simulink model "racing_modes_R2022a"  (R2022a)
settings: Solver=FixedStepAuto  StartTime=0.0  StopTime=10.0  RelTol=1e-3
libraries: simulink x1
settings Model: Creator=no  LastModifiedBy=joser
settings OptimizationCC: DefaultParameterBehavior=Inlined
settings ModelReferenceCC: EnableRefExpFcnMdlSchedulingChecks=off
settings RTWCC: Description=INTECRIO Real-Time Target  SystemTargetFile=irt.tlc  TemplateMakefile=irt_default_tmf
settings STFCustomTargetCC: TargetLangStandard=C99 (ISO)  UtilityFuncGeneration=Shared location  MatFileLogging=on  SystemTargetFile=irt.tlc
settings GRTTargetCC: UtilityFuncGeneration=Shared location  ParMdlRefBuildCompliant=off  CompOptLevelCompliant=off  ConcurrentExecutionCompliant=off  CombineOutputUpdateFcns=off  CPPClassGenCompliant=off  GRTInterface=on  UseToolchainInfoCompliant=off  GenerateASAP2=on

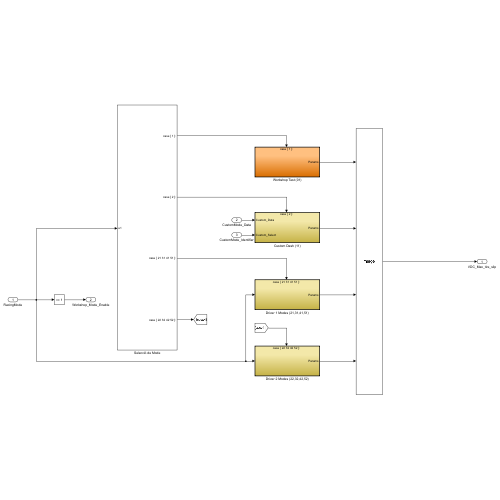
[thumbnail: Simulink's stored preview of the top-level diagram]
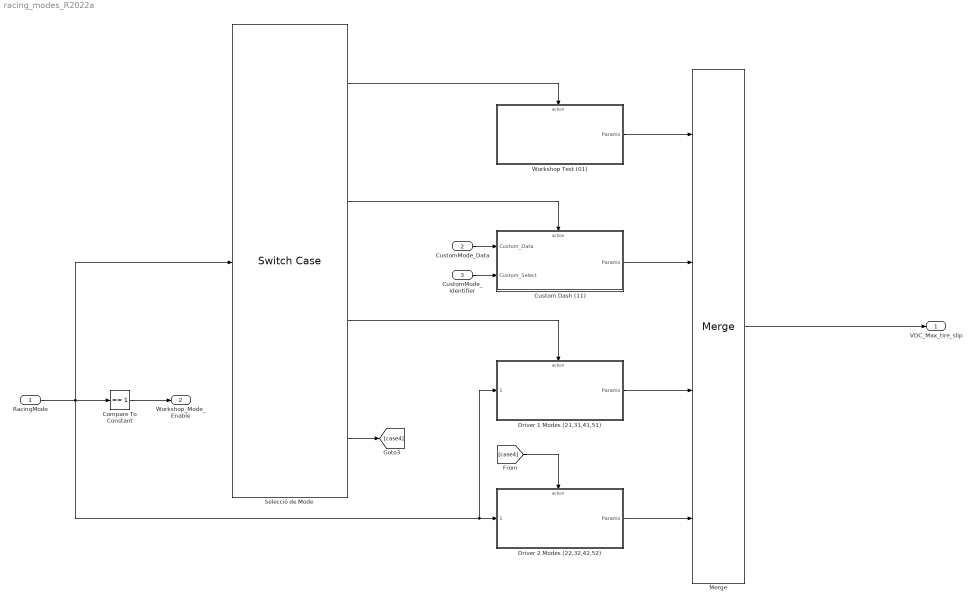
== system racing_modes_R2022a ==
  RacingMode : Inport  OutDataTypeStr=uint8
  CustomMode_Data : Inport  Port=2
  CustomMode_Identifier : Inport  Port=3
  Compare To Constant : simulink/Logic and Bit Operations/Compare To Constant  relop===  const=1  OutDataTypeStr=boolean
  Custom Dash (11) : Subsystem  TreatAsAtomicUnit=on
  Driver 1 Modes (21,31,41,51) : Subsystem  TreatAsAtomicUnit=on
  Driver 2 Modes (22,32,42,52) : Subsystem  TreatAsAtomicUnit=on
  Merge : Merge  Inputs=4
  Selecció de Mode : SwitchCase  CaseConditions={01, 2, [21,31,41,51], [22,32,42,52]}  ShowDefaultCase=off
  Workshop Test (01) : Subsystem  TreatAsAtomicUnit=on
  VDC_Max_tire_slip : Outport
  Workshop_Mode_Enable : Outport  Port=2
  wires:
  CustomMode_Identifier/1 -> Custom Dash (11)/2(Custom_Select)
  Custom Dash (11)/1(Params) -> Merge/2
  RacingMode/1 -> Driver 1 Modes (21,31,41,51)/1(" "), Driver 2 Modes (22,32,42,52)/1(" "), Compare To Constant/1, Selecció de Mode/1
  Workshop Test (01)/1(Params) -> Merge/1
  CustomMode_Data/1 -> Custom Dash (11)/1(Custom_Data)
  Driver 1 Modes (21,31,41,51)/1(Params) -> Merge/3
  Driver 2 Modes (22,32,42,52)/1(Params) -> Merge/4
  Selecció de Mode/4 -> [case4]
  [case4] -> Driver 2 Modes (22,32,42,52)/Action
  Selecció de Mode/1 -> Workshop Test (01)/Action
  Selecció de Mode/2 -> Custom Dash (11)/Action
  Selecció de Mode/3 -> Driver 1 Modes (21,31,41,51)/Action
  Merge/1 -> VDC_Max_tire_slip/1
  Compare To Constant/1 -> Workshop_Mode_Enable/1

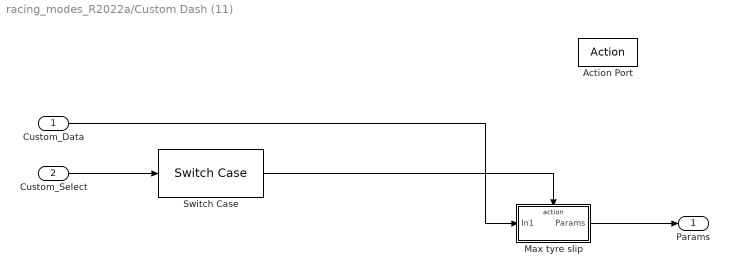
== system racing_modes_R2022a/Custom Dash (11) ==
  Custom_Data : Inport
  Custom_Select : Inport  Port=2
  Action Port : ActionPort  ActionPortLabel=case [ 2 ]:
  Max tyre slip : Subsystem  TreatAsAtomicUnit=on
  Switch Case : SwitchCase  ShowDefaultCase=off
  Params : Outport  VectorParamsAs1DForOutWhenUnconnected=off
  wires:
  Custom_Select/1 -> Switch Case/1
  Custom_Data/1 -> Max tyre slip/1(In1)
  Switch Case/1 -> Max tyre slip/Action
  Max tyre slip/1(Params) -> Params/1

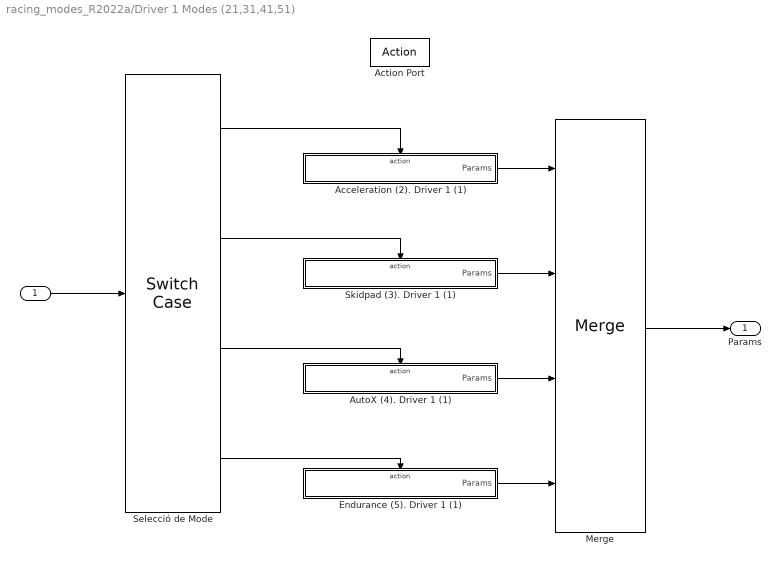
== system racing_modes_R2022a/Driver 1 Modes (21,31,41,51) ==
  " " : Inport  OutDataTypeStr=uint8
  Action Port : ActionPort  ActionPortLabel=case [ 21 31 41 51 ]:
  "Acceleration (2). Driver 1 (1) " : Subsystem  TreatAsAtomicUnit=on
  AutoX (4). Driver 1 (1) : Subsystem  TreatAsAtomicUnit=on
  Endurance (5). Driver 1 (1) : Subsystem  TreatAsAtomicUnit=on
  Merge : Merge  Inputs=4
  Selecció de Mode : SwitchCase  CaseConditions={21,31,41,51}  ShowDefaultCase=off
  Skidpad (3). Driver 1 (1) : Subsystem  TreatAsAtomicUnit=on
  Params : Outport  VectorParamsAs1DForOutWhenUnconnected=off
  wires:
  Merge/1 -> Params/1
  " "/1 -> Selecció de Mode/1
  Selecció de Mode/4 -> Endurance (5). Driver 1 (1)/Action
  Selecció de Mode/3 -> AutoX (4). Driver 1 (1)/Action
  Selecció de Mode/2 -> Skidpad (3). Driver 1 (1)/Action
  Selecció de Mode/1 -> "Acceleration (2). Driver 1 (1) "/Action
  "Acceleration (2). Driver 1 (1) "/1(Params) -> Merge/1
  Skidpad (3). Driver 1 (1)/1(Params) -> Merge/2
  AutoX (4). Driver 1 (1)/1(Params) -> Merge/3
  Endurance (5). Driver 1 (1)/1(Params) -> Merge/4

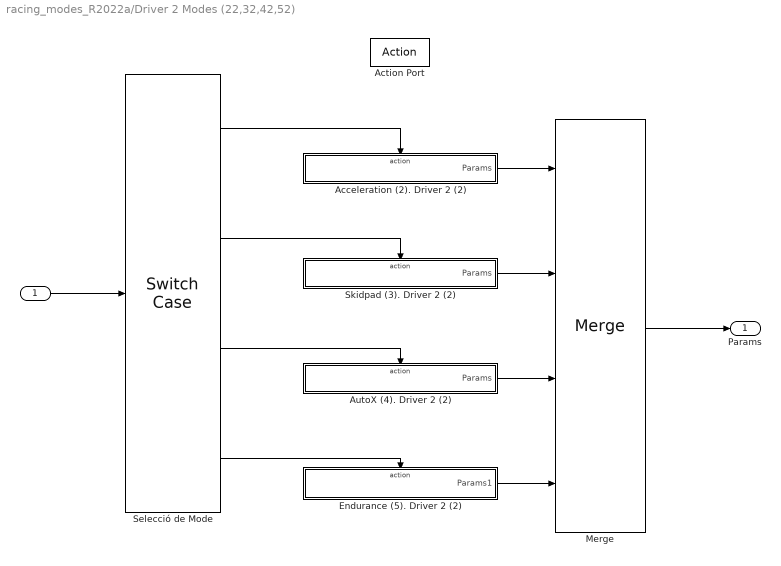
== system racing_modes_R2022a/Driver 2 Modes (22,32,42,52) ==
  " " : Inport  OutDataTypeStr=uint8
  Action Port : ActionPort  ActionPortLabel=case [ 22 32 42 52 ]:
  "Acceleration (2). Driver 2 (2) " : Subsystem  TreatAsAtomicUnit=on
  AutoX (4). Driver 2 (2) : Subsystem  TreatAsAtomicUnit=on
  Endurance (5). Driver 2 (2) : Subsystem  TreatAsAtomicUnit=on
  Merge : Merge  Inputs=4
  Selecció de Mode : SwitchCase  CaseConditions={22,32,42,52}  ShowDefaultCase=off
  Skidpad (3). Driver 2 (2) : Subsystem  TreatAsAtomicUnit=on
  Params : Outport  VectorParamsAs1DForOutWhenUnconnected=off
  wires:
  Merge/1 -> Params/1
  " "/1 -> Selecció de Mode/1
  Selecció de Mode/4 -> Endurance (5). Driver 2 (2)/Action
  Selecció de Mode/3 -> AutoX (4). Driver 2 (2)/Action
  Selecció de Mode/2 -> Skidpad (3). Driver 2 (2)/Action
  Selecció de Mode/1 -> "Acceleration (2). Driver 2 (2) "/Action
  "Acceleration (2). Driver 2 (2) "/1(Params) -> Merge/1
  Skidpad (3). Driver 2 (2)/1(Params) -> Merge/2
  AutoX (4). Driver 2 (2)/1(Params) -> Merge/3
  Endurance (5). Driver 2 (2)/1(Params1) -> Merge/4

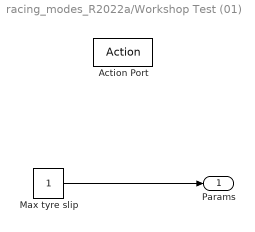
== system racing_modes_R2022a/Workshop Test (01) ==
  Action Port : ActionPort  ActionPortLabel=case [ 1 ]:
  Max tyre slip : Constant
  Params : Outport  VectorParamsAs1DForOutWhenUnconnected=off
  wires:
  Max tyre slip/1 -> Params/1

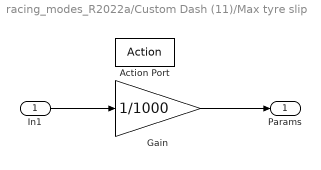
== system racing_modes_R2022a/Custom Dash (11)/Max tyre slip ==
  In1 : Inport
  Action Port : ActionPort
  Gain : Gain  Gain=1/1000
  Params : Outport  VectorParamsAs1DForOutWhenUnconnected=off
  wires:
  In1/1 -> Gain/1
  Gain/1 -> Params/1

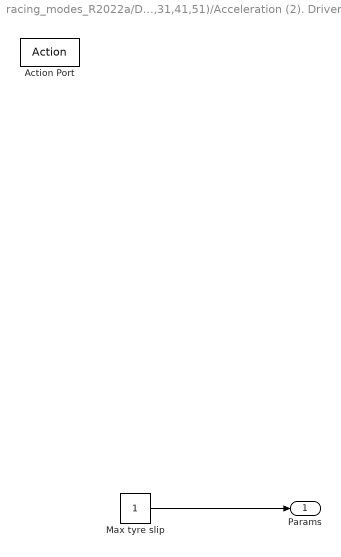
== system racing_modes_R2022a/Driver 1 Modes (21,31,41,51)/Acceleration (2). Driver 1 (1)  ==
  Action Port : ActionPort
  Max tyre slip : Constant
  Params : Outport  VectorParamsAs1DForOutWhenUnconnected=off
  wires:
  Max tyre slip/1 -> Params/1

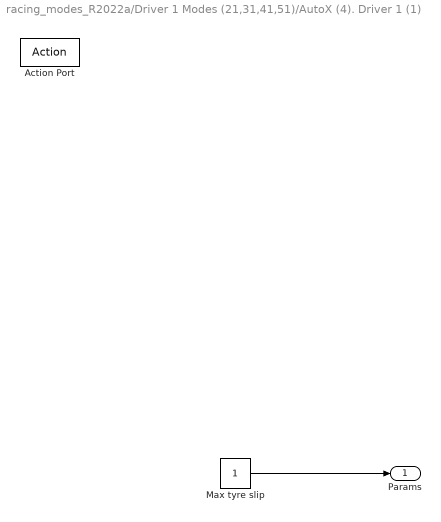
== system racing_modes_R2022a/Driver 1 Modes (21,31,41,51)/AutoX (4). Driver 1 (1) ==
  Action Port : ActionPort
  Max tyre slip : Constant
  Params : Outport  VectorParamsAs1DForOutWhenUnconnected=off
  wires:
  Max tyre slip/1 -> Params/1

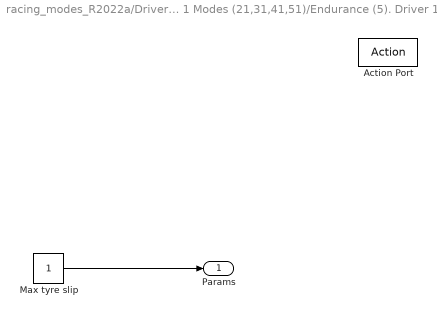
== system racing_modes_R2022a/Driver 1 Modes (21,31,41,51)/Endurance (5). Driver 1 (1) ==
  Action Port : ActionPort
  Max tyre slip : Constant
  Params : Outport  VectorParamsAs1DForOutWhenUnconnected=off
  wires:
  Max tyre slip/1 -> Params/1

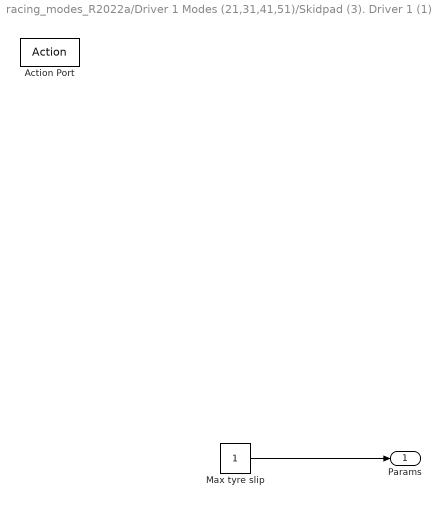
== system racing_modes_R2022a/Driver 1 Modes (21,31,41,51)/Skidpad (3). Driver 1 (1) ==
  Action Port : ActionPort  ActionPortLabel=case [ 31 ]:
  Max tyre slip : Constant
  Params : Outport  VectorParamsAs1DForOutWhenUnconnected=off
  wires:
  Max tyre slip/1 -> Params/1

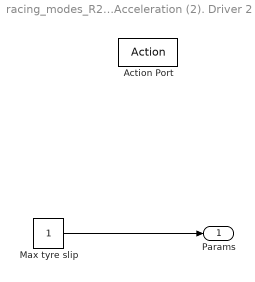
== system racing_modes_R2022a/Driver 2 Modes (22,32,42,52)/Acceleration (2). Driver 2 (2)  ==
  Action Port : ActionPort
  Max tyre slip : Constant
  Params : Outport  VectorParamsAs1DForOutWhenUnconnected=off
  wires:
  Max tyre slip/1 -> Params/1

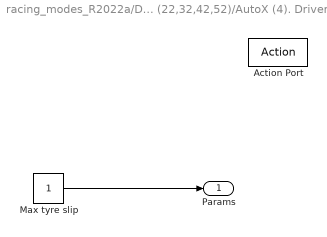
== system racing_modes_R2022a/Driver 2 Modes (22,32,42,52)/AutoX (4). Driver 2 (2) ==
  Action Port : ActionPort
  Max tyre slip : Constant
  Params : Outport  VectorParamsAs1DForOutWhenUnconnected=off
  wires:
  Max tyre slip/1 -> Params/1

== system racing_modes_R2022a/Driver 2 Modes (22,32,42,52)/Endurance (5). Driver 2 (2) ==
  Action Port : ActionPort
  Max tyre slip1 : Constant
  Params1 : Outport  VectorParamsAs1DForOutWhenUnconnected=off
  wires:
  Max tyre slip1/1 -> Params1/1

== system racing_modes_R2022a/Driver 2 Modes (22,32,42,52)/Skidpad (3). Driver 2 (2) ==
  Action Port : ActionPort  ActionPortLabel=case [ 32 ]:
  Max tyre slip : Constant
  Params : Outport  VectorParamsAs1DForOutWhenUnconnected=off
  wires:
  Max tyre slip/1 -> Params/1
